simulink model "Two_FSK"  (R2013a)
settings: Solver=ode45  StartTime=0.0  StopTime=10.0  RelTol=1e-3
libraries: dsparch4 x4, commrandsrc2 x1, commsrccod2 x1
settings Model: Creator=sliencer  LastModifiedBy=sliencer

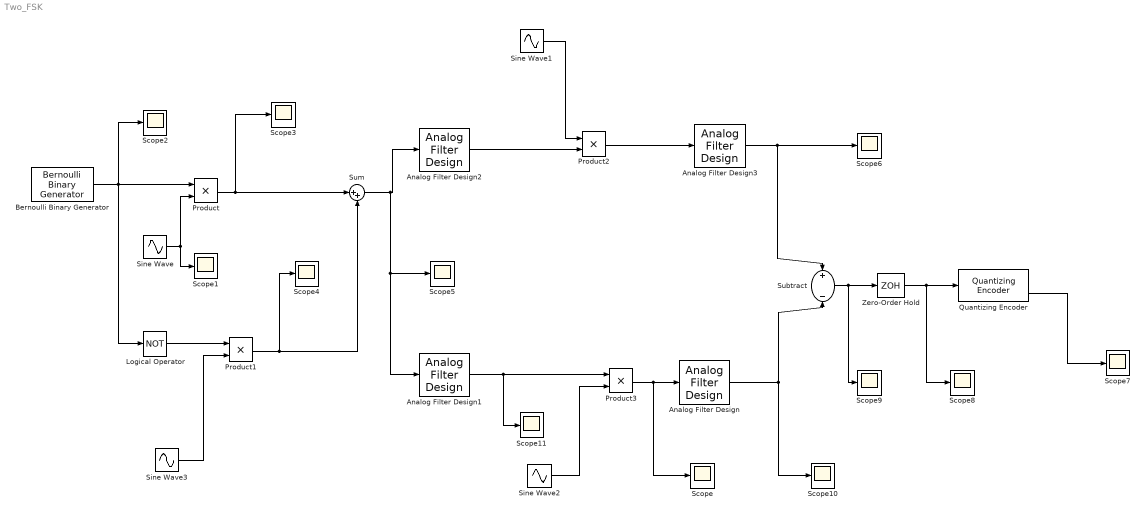
== system Two_FSK ==
  Analog Filter Design : dsparch4/Analog Filter Design  method=Butterworth  filttype=Lowpass  N=8  Wlo=20  Whi=80  Rp=2  Rs=40
  Analog Filter Design1 : dsparch4/Analog Filter Design  method=Butterworth  filttype=Bandpass  N=8  Wlo=10*pi  Whi=30*pi  Rp=2  Rs=40
  Analog Filter Design2 : dsparch4/Analog Filter Design  method=Butterworth  filttype=Bandpass  N=8  Wlo=60*pi  Whi=100*pi  Rp=2  Rs=40
  Analog Filter Design3 : dsparch4/Analog Filter Design  method=Butterworth  filttype=Lowpass  N=8  Wlo=80  Whi=80  Rp=2  Rs=40
  Bernoulli Binary Generator : commrandsrc2/Bernoulli Binary Generator  P=0.5  seed=61  Ts=1  frameBased=off  sampPerFrame=1  orient=off  outDataType=double
  Logical Operator : Logic  Operator=NOT  AllPortsSameDT=off  OutDataTypeStr=boolean
  Product{,1..3} (4 alike) : Product
  Quantizing Encoder : commsrccod2/Quantizing Encoder  partition=[0.2]  codebook=[0 1]  idxDType=double
  Scope{,1..11} (12 alike) : Scope
      Scope10 settings: SaveName=ScopeData10
      Scope11 settings: SaveName=ScopeData11
      Scope2 settings: SaveName=ScopeData2
      Scope3 settings: SaveName=ScopeData3
      Scope4 settings: SaveName=ScopeData4
      Scope5 settings: SaveName=ScopeData5
      Scope6 settings: SaveName=ScopeData6
      Scope7 settings: SaveName=ScopeData7
      Scope8 settings: SaveName=ScopeData8
      Scope9 settings: SaveName=ScopeData9
  Sine Wave : Sin  Frequency=80*pi  SampleTime=1/500
  Sine Wave1 : Sin  Frequency=80*pi  SampleTime=1/500
  Sine Wave2 : Sin  Frequency=80*pi  SampleTime=1/500
  Sine Wave3 : Sin  Frequency=20*pi  SampleTime=1/500
  Subtract : Sum  Inputs=+-  SampleTime=1
  Sum : Sum  Inputs=|++
  Zero-Order Hold : ZeroOrderHold
  wires:
  Bernoulli Binary Generator/1 -> Logical Operator/1, Scope2/1, Product/1
  Sine Wave/1 -> Scope1/1, Product/2
  Product/1 -> Scope3/1, Sum/1
  Logical Operator/1 -> Product1/1
  Product1/1 -> Scope4/1, Sum/2
  Sum/1 -> Scope5/1, Analog Filter Design1/1, Analog Filter Design2/1
  Product2/1 -> Analog Filter Design3/1
  Analog Filter Design2/1 -> Product2/2
  Sine Wave1/1 -> Product2/1
  Analog Filter Design3/1 -> Scope6/1, Subtract/1
  Subtract/1 -> Scope9/1, Zero-Order Hold/1
  Zero-Order Hold/1 -> Scope8/1, Quantizing Encoder/1
  Quantizing Encoder/2 -> Scope7/1
  Analog Filter Design1/1 -> Scope11/1, Product3/1
  Sine Wave2/1 -> Product3/2
  Product3/1 -> Scope/1, Analog Filter Design/1
  Analog Filter Design/1 -> Scope10/1, Subtract/2
  Sine Wave3/1 -> Product1/2
